simulink subsystem "Throttle_and_Manifold"  (R2024b)
settings: Solver=VariableStepAuto  StartTime=0.0  StopTime=10.0  RelTol=1e-3
settings Model: Creator=The MathWorks, Inc.  LastModifiedBy=The MathWorks, Inc.

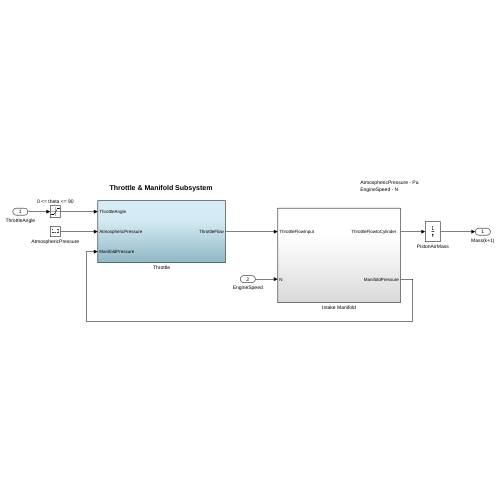
[thumbnail: Simulink's stored preview of the top-level diagram]
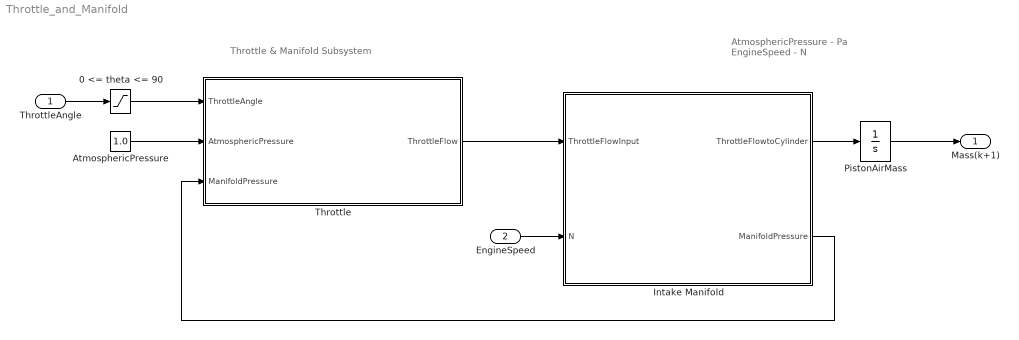
== system Throttle_and_Manifold ==
  note: AtmosphericPressure - Pa
      | EngineSpeed - N
  note: Throttle & Manifold Subsystem
  ThrottleAngle : Inport  Unit=deg
  EngineSpeed : Inport  Port=2
  0 <= theta <= 90 : Saturate  UpperLimit=90  LowerLimit=0
  AtmosphericPressure : Constant  Value=1.0
  Intake Manifold : Subsystem
  PistonAirMass : Integrator
  Throttle : Subsystem
  Mass(k+1) : Outport  InitialOutput=0  VectorParamsAs1DForOutWhenUnconnected=off
  wires:
  0 <= theta <= 90/1 -> Throttle/1(ThrottleAngle)
  ThrottleAngle/1 -> 0 <= theta <= 90/1
  Throttle/1(ThrottleFlow) -> Intake Manifold/1(ThrottleFlowInput)
  EngineSpeed/1 -> Intake Manifold/2(N)
  Intake Manifold/2(ManifoldPressure) -> Throttle/3(ManifoldPressure)
  AtmosphericPressure/1 -> Throttle/2("AtmosphericPressure ")
  Intake Manifold/1("ThrottleFlowtoCylinder ") -> PistonAirMass/1
  PistonAirMass/1 -> Mass(k+1)/1

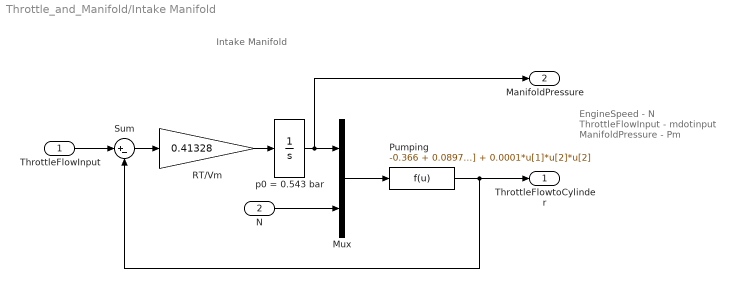
== system Throttle_and_Manifold/Intake Manifold ==
  note: Intake Manifold
  note: EngineSpeed - N
      | ThrottleFlowInput - mdotinput
      | ManifoldPressure - Pm
  ThrottleFlowInput : Inport
  N : Inport  Port=2  Unit=rad/sec
  Mux : Mux  Inputs=2
  Pumping : Fcn  Expr=-0.366 + 0.08979*u[1]*u[2] - 0.0337*u[2]*u[1]*u[1] + 0.0001*u[1]*u[2]*u[2]
  RT/Vm : Gain  Gain=0.41328  SaturateOnIntegerOverflow=on  OutDataTypeStr=Inherit: Same as input  ParamDataTypeStr=Inherit: Same as input
  Sum : Sum  Inputs=|+-  InputSameDT=on  SaturateOnIntegerOverflow=on  OutDataTypeStr=Inherit: Same as first input
  p0 = 0.543 bar : Integrator  InitialCondition=.543
  "ThrottleFlowtoCylinder " : Outport  Unit=g/s  InitialOutput=0  VectorParamsAs1DForOutWhenUnconnected=off
  ManifoldPressure : Outport  Port=2  InitialOutput=0  VectorParamsAs1DForOutWhenUnconnected=off
  wires:
  Pumping/1 -> "ThrottleFlowtoCylinder "/1, Sum/2
  Sum/1 -> RT/Vm/1
  p0 = 0.543 bar/1 -> ManifoldPressure/1, Mux/1
  Mux/1 -> Pumping/1
  N/1 -> Mux/2
  RT/Vm/1 -> p0 = 0.543 bar/1
  ThrottleFlowInput/1 -> Sum/1

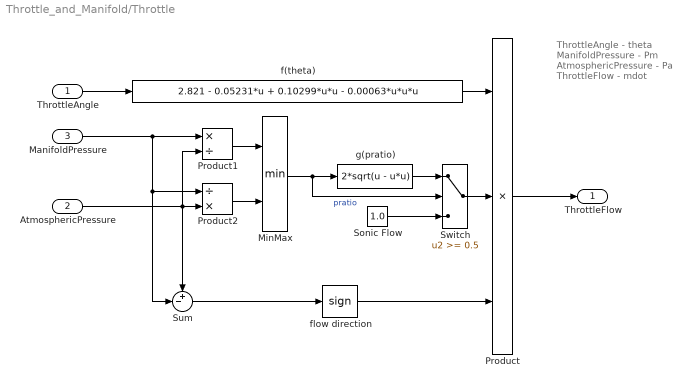
== system Throttle_and_Manifold/Throttle ==
  note: ThrottleAngle - theta
      | ManifoldPressure - Pm
      | AtmosphericPressure - Pa
      | ThrottleFlow - mdot
  ThrottleAngle : Inport  Unit=deg
  "AtmosphericPressure " : Inport  Port=2  Unit=bar
  ManifoldPressure : Inport  Port=3  Unit=bar
  MinMax : MinMax  Inputs=2  InputSameDT=on  SaturateOnIntegerOverflow=on
  Product : Product  Inputs=3  InputSameDT=on  RndMeth=Zero  SaturateOnIntegerOverflow=on  OutDataTypeStr=Inherit: Same as first input
  Product1 : Product  Inputs=*/  InputSameDT=on  RndMeth=Zero  SaturateOnIntegerOverflow=on  OutDataTypeStr=Inherit: Same as first input
  Product2 : Product  Inputs=/*  InputSameDT=on  RndMeth=Zero  SaturateOnIntegerOverflow=on  OutDataTypeStr=Inherit: Same as first input
  "Sonic Flow " : Constant  Value=1.0
  Sum : Sum  Inputs=+-|  InputSameDT=on  SaturateOnIntegerOverflow=on  OutDataTypeStr=Inherit: Same as first input
  Switch : Switch  Threshold=0.5
  f(theta) : Fcn  Expr=2.821 - 0.05231*u + 0.10299*u*u - 0.00063*u*u*u
  flow direction : Signum
  g(pratio) : Fcn  Expr=2*sqrt(u - u*u)
  ThrottleFlow : Outport  Unit=g/s  InitialOutput=0  VectorParamsAs1DForOutWhenUnconnected=off
  wires:
  f(theta)/1 -> Product/1
  Product/1 -> ThrottleFlow/1
  ThrottleAngle/1 -> f(theta)/1
  MinMax/1 -> g(pratio)/1, Switch/2  "pratio"
  Sum/1 -> flow direction/1
  flow direction/1 -> Product/3
  Switch/1 -> Product/2
  "Sonic Flow "/1 -> Switch/3
  g(pratio)/1 -> Switch/1
  "AtmosphericPressure "/1 -> Product2/2, Sum/1, Product1/2
  Product1/1 -> MinMax/1
  Product2/1 -> MinMax/2
  ManifoldPressure/1 -> Product1/1, Product2/1, Sum/2
